simulink library "INP_EMFR"  (R2022a)
settings: Solver=VariableStepAuto  StartTime=0.0  StopTime=10.0  RelTol=1e-3
settings Model: Creator=blatak  LastModifiedBy=blatak

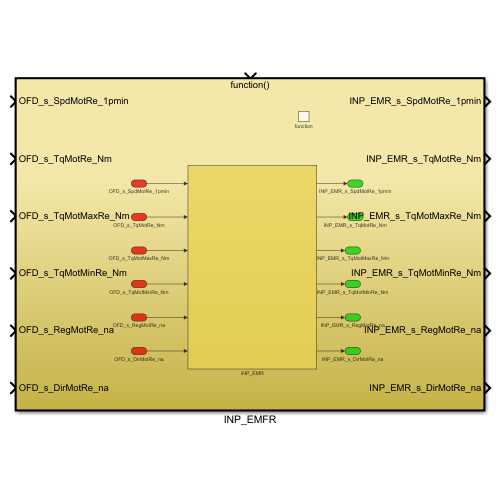
[thumbnail: Simulink's stored preview of the top-level diagram]
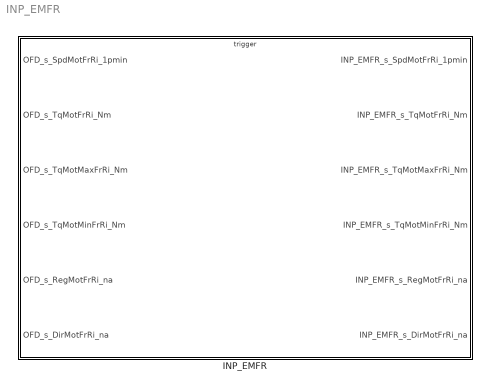
== system INP_EMFR ==
  INP_EMFR : Subsystem  TreatAsAtomicUnit=on

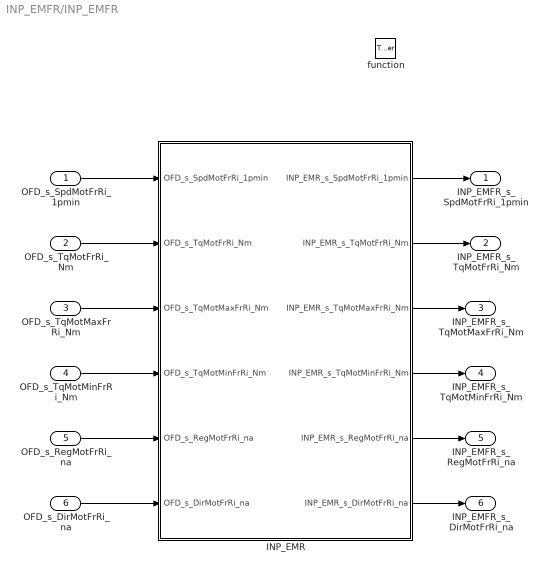
== system INP_EMFR/INP_EMFR ==
  OFD_s_SpdMotFrRi_1pmin : Inport
  OFD_s_TqMotFrRi_Nm : Inport  Port=2
  OFD_s_TqMotMaxFrRi_Nm : Inport  Port=3
  OFD_s_TqMotMinFrRi_Nm : Inport  Port=4
  OFD_s_RegMotFrRi_na : Inport  Port=5
  OFD_s_DirMotFrRi_na : Inport  Port=6
  function : TriggerPort  TriggerType=function-call  VariantControl=(inherit)
  INP_EMR : Subsystem
  INP_EMFR_s_SpdMotFrRi_1pmin : Outport
  INP_EMFR_s_TqMotFrRi_Nm : Outport  Port=2
  INP_EMFR_s_TqMotMaxFrRi_Nm : Outport  Port=3
  INP_EMFR_s_TqMotMinFrRi_Nm : Outport  Port=4
  INP_EMFR_s_RegMotFrRi_na : Outport  Port=5
  INP_EMFR_s_DirMotFrRi_na : Outport  Port=6
  wires:
  OFD_s_TqMotFrRi_Nm/1 -> INP_EMR/2(OFD_s_TqMotFrRi_Nm)
  OFD_s_SpdMotFrRi_1pmin/1 -> INP_EMR/1(OFD_s_SpdMotFrRi_1pmin)
  INP_EMR/1(INP_EMR_s_SpdMotFrRi_1pmin) -> INP_EMFR_s_SpdMotFrRi_1pmin/1
  INP_EMR/2(INP_EMR_s_TqMotFrRi_Nm) -> INP_EMFR_s_TqMotFrRi_Nm/1
  OFD_s_TqMotMaxFrRi_Nm/1 -> INP_EMR/3(OFD_s_TqMotMaxFrRi_Nm)
  OFD_s_TqMotMinFrRi_Nm/1 -> INP_EMR/4(OFD_s_TqMotMinFrRi_Nm)
  OFD_s_RegMotFrRi_na/1 -> INP_EMR/5(OFD_s_RegMotFrRi_na)
  OFD_s_DirMotFrRi_na/1 -> INP_EMR/6(OFD_s_DirMotFrRi_na)
  INP_EMR/3(INP_EMR_s_TqMotMaxFrRi_Nm) -> INP_EMFR_s_TqMotMaxFrRi_Nm/1
  INP_EMR/4(INP_EMR_s_TqMotMinFrRi_Nm) -> INP_EMFR_s_TqMotMinFrRi_Nm/1
  INP_EMR/5(INP_EMR_s_RegMotFrRi_na) -> INP_EMFR_s_RegMotFrRi_na/1
  INP_EMR/6(INP_EMR_s_DirMotFrRi_na) -> INP_EMFR_s_DirMotFrRi_na/1

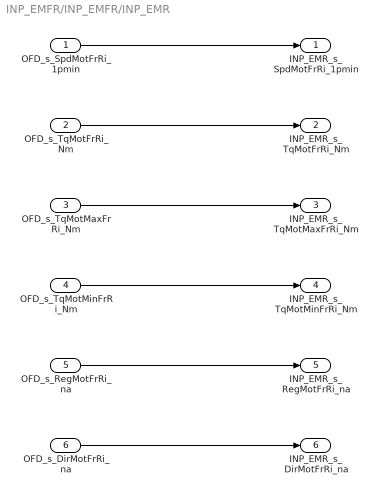
== system INP_EMFR/INP_EMFR/INP_EMR ==
  OFD_s_SpdMotFrRi_1pmin : Inport
  OFD_s_TqMotFrRi_Nm : Inport  Port=2
  OFD_s_TqMotMaxFrRi_Nm : Inport  Port=3
  OFD_s_TqMotMinFrRi_Nm : Inport  Port=4
  OFD_s_RegMotFrRi_na : Inport  Port=5
  OFD_s_DirMotFrRi_na : Inport  Port=6
  INP_EMR_s_SpdMotFrRi_1pmin : Outport
  INP_EMR_s_TqMotFrRi_Nm : Outport  Port=2
  INP_EMR_s_TqMotMaxFrRi_Nm : Outport  Port=3
  INP_EMR_s_TqMotMinFrRi_Nm : Outport  Port=4
  INP_EMR_s_RegMotFrRi_na : Outport  Port=5
  INP_EMR_s_DirMotFrRi_na : Outport  Port=6
  wires:
  OFD_s_TqMotFrRi_Nm/1 -> INP_EMR_s_TqMotFrRi_Nm/1
  OFD_s_SpdMotFrRi_1pmin/1 -> INP_EMR_s_SpdMotFrRi_1pmin/1
  OFD_s_TqMotMinFrRi_Nm/1 -> INP_EMR_s_TqMotMinFrRi_Nm/1
  OFD_s_TqMotMaxFrRi_Nm/1 -> INP_EMR_s_TqMotMaxFrRi_Nm/1
  OFD_s_DirMotFrRi_na/1 -> INP_EMR_s_DirMotFrRi_na/1
  OFD_s_RegMotFrRi_na/1 -> INP_EMR_s_RegMotFrRi_na/1
